simulink model "trimming"  (R2020a)
settings: Solver=VariableStepAuto  StartTime=0.0  StopTime=10.0  RelTol=1e-3
values from neighbouring files (symbols this model uses):
  g = 32.17    [PreLoadFcn.m]
  state0 = [IC.npos IC.epos IC.alt IC.q0 IC.q1 IC.q2 IC.q3  IC.p IC.q IC.r IC.alpha IC.beta IC.mu IC.Vt IC.chi IC.gamma]    [PreLoadFcn.m]
undefined symbols (not defined in the file or in its folder): Aactuator, ac, AeroCoeff, ft, kg, m, Newton, Raphson, s, slug
libraries: aerolibconvert2 x9, simulink x2
(part 1 of 2)
settings Model: Creator=User  LastModifiedBy=user

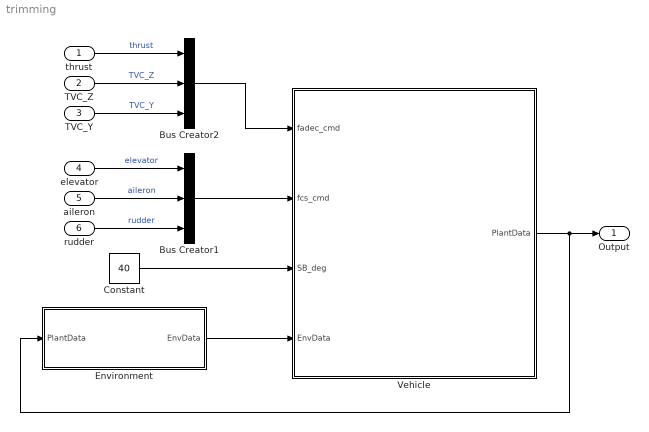
== system trimming ==
  thrust : Inport
  TVC_Z : Inport  Port=2
  TVC_Y : Inport  Port=3
  elevator : Inport  Port=4
  aileron : Inport  Port=5
  rudder : Inport  Port=6
  Bus Creator1 : BusCreator  Inputs=3
  Bus Creator2 : BusCreator  Inputs=3
  Constant : Constant  Value=40
  Environment : Subsystem
      mask Display:
      | image('aeroenvironment.bmp','center')
      | port_label('input',1,'PlantData')
      | port_label('output',1,'EnvData')
  Vehicle : Subsystem
  Output : Outport
  wires:
  Environment/1(EnvData) -> Vehicle/4(EnvData)
  Constant/1 -> Vehicle/3(" SB_deg")
  Vehicle/1(PlantData) -> Environment/1(PlantData), Output/1
  Bus Creator2/1 -> Vehicle/1(fadec_cmd)
  TVC_Y/1 -> Bus Creator2/3  "TVC_Y"
  TVC_Z/1 -> Bus Creator2/2  "TVC_Z"
  thrust/1 -> Bus Creator2/1  "thrust"
  elevator/1 -> Bus Creator1/1  "elevator"
  rudder/1 -> Bus Creator1/3  "rudder"
  aileron/1 -> Bus Creator1/2  "aileron"
  Bus Creator1/1 -> Vehicle/2(fcs_cmd)

== system trimming/Environment ==
  PlantData : Inport
  "ISP " : Subsystem
  end5 : Terminator
  end8 : Terminator
  end9 : Terminator
  gravity (ft/s^2) : Constant  Value=g
  Out Bus Element : Outport  PortName=EnvData  Element=P
  Out Bus Element1 : Outport  PortName=EnvData  Element=AirDensity
  Out Bus Element2 : Outport  PortName=EnvData  Element=qbar
  Out Bus Element3 : Outport  PortName=EnvData  Element=Mach
  Out Bus Element4 : Outport  PortName=EnvData  Element=g
  wires:
  "ISP "/7(mu) -> end9/1
  "ISP "/5(T(K)) -> end5/1
  "ISP "/6(g (m/s^2)) -> end8/1
  PlantData/1 -> "ISP "/1(PlantData)
  "ISP "/1(P(HPa)) -> Out Bus Element/1
  "ISP "/2(rho(kg/m^3)) -> Out Bus Element1/1
  "ISP "/3(qbar (lbf/ft^2)) -> Out Bus Element2/1
  "ISP "/4("Mach ") -> Out Bus Element3/1
  gravity (ft/s^2)/1 -> Out Bus Element4/1  "g"

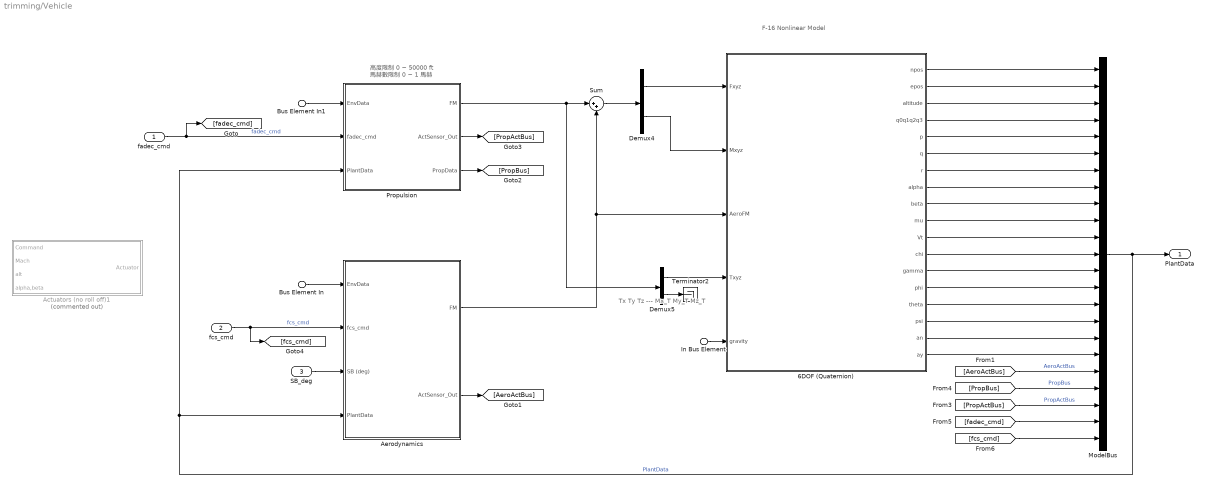
== system trimming/Vehicle ==
  note: F-16 Nonlinear Model
  note: Tx
      | Ty
      | Tz
      | ---
      | Mx_T
      | My_T
      | Mz_T
  note: 高度限制 0 ~ 50000 ft
      | 馬赫數限制 0 ~ 1 馬赫
  fadec_cmd : Inport
  fcs_cmd : Inport  Port=2
  " SB_deg" : Inport  Port=3
  Bus Element In : Inport  Port=4  PortName=EnvData
  Bus Element In1 : Inport  Port=4  PortName=EnvData
  In Bus Element : Inport  Port=4  PortName=EnvData  Element=g
  6DOF (Quaternion) : Subsystem
  Actuators (no roll off)1 : Subsystem  Commented=on
  Aerodynamics : Subsystem
  Demux4 : Demux  Outputs=[3, 3]
  Demux5 : Demux  Outputs=[3, 3]
  ModelBus : BusCreator  Inputs=23
  Propulsion : Subsystem
  Sum : Sum  Inputs=|++
  Terminator2 : Terminator
  PlantData : Outport
  wires:
  6DOF (Quaternion)/4(q0q1q2q3) -> ModelBus/4
  6DOF (Quaternion)/11(Vt) -> ModelBus/11
  6DOF (Quaternion)/3(altitude) -> ModelBus/3
  ModelBus/1 -> Aerodynamics/4(PlantData), Propulsion/3(PlantData), PlantData/1  "PlantData"
  6DOF (Quaternion)/1(npos) -> ModelBus/1
  6DOF (Quaternion)/2(epos) -> ModelBus/2
  " SB_deg"/1 -> Aerodynamics/3(" SB (deg)")
  Aerodynamics/1(FM) -> Sum/2, 6DOF (Quaternion)/3(AeroFM)
  Aerodynamics/2(ActSensor_Out) -> [AeroActBus]
  Propulsion/1(FM) -> Demux5/1, Sum/1
  fcs_cmd/1 -> [fcs_cmd], Aerodynamics/2(fcs_cmd)  "fcs_cmd"
  fadec_cmd/1 -> Propulsion/2(fadec_cmd), [fadec_cmd]  "fadec_cmd"
  Propulsion/2(ActSensor_Out) -> [PropActBus]
  Propulsion/3(PropData) -> [PropBus]
  Sum/1 -> Demux4/1
  Demux4/2 -> 6DOF (Quaternion)/2(Mxyz)
  Demux4/1 -> 6DOF (Quaternion)/1(Fxyz)
  Demux5/1 -> 6DOF (Quaternion)/4(Txyz)
  Demux5/2 -> Terminator2/1
  In Bus Element/1 -> 6DOF (Quaternion)/5(gravity)
  6DOF (Quaternion)/17(an) -> ModelBus/17
  6DOF (Quaternion)/18(ay) -> ModelBus/18
  6DOF (Quaternion)/5(p) -> ModelBus/5
  6DOF (Quaternion)/6(q) -> ModelBus/6
  6DOF (Quaternion)/7(r) -> ModelBus/7
  6DOF (Quaternion)/8(alpha) -> ModelBus/8
  6DOF (Quaternion)/9(beta) -> ModelBus/9
  6DOF (Quaternion)/10(mu) -> ModelBus/10
  6DOF (Quaternion)/12(chi) -> ModelBus/12
  6DOF (Quaternion)/13(gamma) -> ModelBus/13
  6DOF (Quaternion)/14(phi) -> ModelBus/14
  6DOF (Quaternion)/15(theta) -> ModelBus/15
  6DOF (Quaternion)/16(psi) -> ModelBus/16
  Bus Element In/1 -> Aerodynamics/1(EnvData)
  Bus Element In1/1 -> Propulsion/1(EnvData)
  [PropActBus] -> ModelBus/21  "PropActBus"
  [AeroActBus] -> ModelBus/19  "AeroActBus"
  [PropBus] -> ModelBus/20  "PropBus"
  [fadec_cmd] -> ModelBus/22
  [fcs_cmd] -> ModelBus/23

== system trimming/Environment/ISP  ==
  note: 1 T
      | 2 a (Speed of sound)
      | 3 P
      | 4 rho
      | 5 g
      | 6 mu (Coefficient of viscosity)
  In Bus Element : Inport  PortName=PlantData  Element=Vt
  In Bus Element1 : Inport  PortName=PlantData  Element=altitude
  Demux : Demux  Outputs=[1,1,1,1,1,1]
      settings: DisplayOption=none
  Density Conversion : aerolibconvert2/Density Conversion  IU=kg/m^3  OU=slug/ft^3
      settings: SourceProductBaseCode=AE
  Divide1 : Product  Inputs=*/
  Length Conversion : aerolibconvert2/Length Conversion  IU=ft  OU=m
  MATLAB Function : MATLAB Function  TreatAsAtomicUnit=on
  Product : Product
  Square : Math  Operator=square  SignedPower=on  SaturateOnIntegerOverflow=on
  Velocity Conversion : aerolibconvert2/Velocity Conversion  IU=m/s  OU=ft/s
  r2d1 : Gain  Gain=0.5  SaturateOnIntegerOverflow=on  OutDataTypeStr=Inherit: Same as input  ParamDataTypeStr=Inherit: Same as input
  r2d2 : Gain  Gain=-1  SaturateOnIntegerOverflow=on  OutDataTypeStr=Inherit: Same as input  ParamDataTypeStr=Inherit: Same as input
  P(HPa) : Outport  VectorParamsAs1DForOutWhenUnconnected=off
  rho(kg/m^3) : Outport  Port=2  VectorParamsAs1DForOutWhenUnconnected=off
  qbar (lbf/ft^2) : Outport  Port=3  VectorParamsAs1DForOutWhenUnconnected=off
  "Mach " : Outport  Port=4  VectorParamsAs1DForOutWhenUnconnected=off
  T(K) : Outport  Port=5  VectorParamsAs1DForOutWhenUnconnected=off
  g (m/s^2) : Outport  Port=6  VectorParamsAs1DForOutWhenUnconnected=off
  mu : Outport  Port=7  VectorParamsAs1DForOutWhenUnconnected=off
  wires:
  MATLAB Function/1(ISP_output) -> Demux/1
  Length Conversion/1 -> MATLAB Function/1(h)
  Velocity Conversion/1 -> Divide1/2
  Density Conversion/1 -> Product/2  "rho(slugs/ft^3)"
  Demux/4 -> Density Conversion/1, rho(kg/m^3)/1  "rho(kg/m^3)"
  Demux/2 -> Velocity Conversion/1  "a(m/s)"
  Demux/1 -> T(K)/1  "T(K)"
  Divide1/1 -> "Mach "/1
  Demux/5 -> g (m/s^2)/1  "g (m/s^2)"
  Demux/6 -> mu/1  "mu"
  Product/1 -> r2d1/1
  Square/1 -> Product/1
  In Bus Element/1 -> Divide1/1, Square/1  "Vt (ft/s)"
  Demux/3 -> P(HPa)/1  "P(Pa)"
  r2d2/1 -> Length Conversion/1  "H(ft)"
  r2d1/1 -> qbar (lbf/ft^2)/1  "qbar (lbf/ft^2)"
  In Bus Element1/1 -> r2d2/1

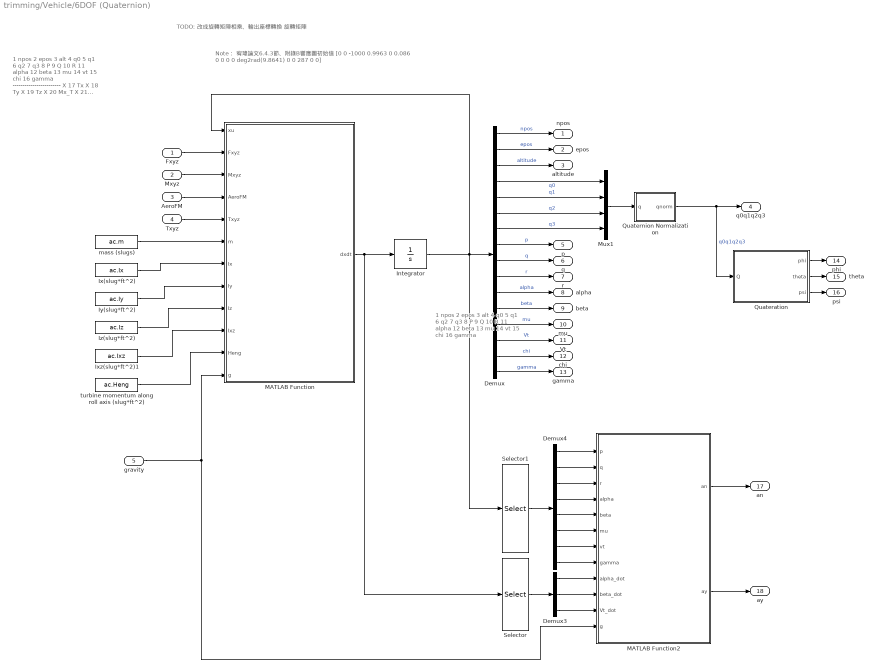
== system trimming/Vehicle/6DOF (Quaternion) ==
  note: TODO: 改成旋轉矩陣相乘、輸出座標轉換 旋轉矩陣
  note: 1 npos
      | 2 epos
      | 3 alt
      | 4 q0
      | 5 q1
      | 6 q2
      | 7 q3
      | 8 P
      | 9 Q
      | 10 R
      | 11 alpha
      | 12 beta
      | 13 mu
      | 14 vt
      | 15 chi
      | 16 gamma
      | ------------------------
      | X 17 Tx
      | X 18 Ty
      | X 19 Tz
      | X 20 Mx_T
      | X 21 My_T
      | X 22 Mz_T
      | X 23 T
      | --------------------
      | X 24 ele
      | X 25 ail
      | X 26 rud
      | -------------------
      | X 27 delta_z
      | X 28 delta_y
      | -----------------
      | X 29 qbar
      | -----------------
      | X 30 CXT
      | X 31 CYT
      | X 32 CZT
      | X 33 CLT
      | X 34 CMT
      | X 35 CNT
      | -----------------
      | X 36 lef
  note: 1 npos
      | 2 epos
      | 3 alt
      | 4 q0
      | 5 q1
      | 6 q2
      | 7 q3
      | 8 P
      | 9 Q
      | 10 R
      | 11 alpha
      | 12 beta
      | 13 mu
      | 14 vt
      | 15 chi
      | 16 gamma
  note: Note：
      |
      | 宥瑋論文6.4.3節、附錄B響應圖初始值
      | [0 0 -1000 0.9963 0 0.086 0  0 0 0 deg2rad(9.8641) 0 0 287 0 0]
  Fxyz : Inport
  Mxyz : Inport  Port=2
  AeroFM : Inport  Port=3
  Txyz : Inport  Port=4
  gravity : Inport  Port=5
  Demux : Demux  Outputs=16
      settings: DisplayOption=none
  Demux3 : Demux  Outputs=3
  Demux4 : Demux  Outputs=8
  Integrator : Integrator  InitialCondition=state0
  Ix(slug*ft^2) : Constant  Value=ac.Ix
  Ixz(slug*ft^2)1 : Constant  Value=ac.Ixz
  Iy(slug*ft^2) : Constant  Value=ac.Iy
  Iz(slug*ft^2) : Constant  Value=ac.Iz
  MATLAB Function : MATLAB Function  TreatAsAtomicUnit=on
  MATLAB Function2 : MATLAB Function  TreatAsAtomicUnit=on
  Mux1 : Mux  Inputs=[1,1,1,1]
  Quateration : MATLAB Function  TreatAsAtomicUnit=on
  Quaternion Normalization : Subsystem
  Selector : Selector  InputPortWidth=16  IndexOptions=Index vector (dialog)  Indices=[11 12 14]  OutputSizes=3
  Selector1 : Selector  InputPortWidth=16  IndexOptions=Index vector (dialog)  Indices=[8:14 16]  OutputSizes=3
  mass (slugs) : Constant  Value=ac.m
  turbine momentum along roll axis (slug*ft^2) : Constant  Value=ac.Heng
  npos : Outport  VectorParamsAs1DForOutWhenUnconnected=off
  epos : Outport  Port=2  VectorParamsAs1DForOutWhenUnconnected=off
  altitude : Outport  Port=3  VectorParamsAs1DForOutWhenUnconnected=off
  q0q1q2q3 : Outport  Port=4
  p : Outport  Port=5  VectorParamsAs1DForOutWhenUnconnected=off
  q : Outport  Port=6  VectorParamsAs1DForOutWhenUnconnected=off
  r : Outport  Port=7  VectorParamsAs1DForOutWhenUnconnected=off
  alpha : Outport  Port=8  VectorParamsAs1DForOutWhenUnconnected=off
  beta : Outport  Port=9  VectorParamsAs1DForOutWhenUnconnected=off
  mu : Outport  Port=10  VectorParamsAs1DForOutWhenUnconnected=off
  Vt : Outport  Port=11  VectorParamsAs1DForOutWhenUnconnected=off
  chi : Outport  Port=12  VectorParamsAs1DForOutWhenUnconnected=off
  gamma : Outport  Port=13  VectorParamsAs1DForOutWhenUnconnected=off
  phi : Outport  Port=14  VectorParamsAs1DForOutWhenUnconnected=off
  theta : Outport  Port=15  VectorParamsAs1DForOutWhenUnconnected=off
  psi : Outport  Port=16  VectorParamsAs1DForOutWhenUnconnected=off
  an : Outport  Port=17
  ay : Outport  Port=18
  wires:
  Demux/2 -> epos/1  "epos"
  Demux/3 -> altitude/1  "altitude"
  Integrator/1 -> MATLAB Function/1(xu), Selector1/1, Demux/1
  MATLAB Function/1(dxdt) -> Integrator/1, Selector/1
  Demux/1 -> npos/1  "npos"
  Demux/5 -> Mux1/2  "q1"
  Demux/4 -> Mux1/1  "q0"
  Demux/7 -> Mux1/4  "q3"
  Demux/6 -> Mux1/3  "q2"
  Demux/8 -> p/1  "p"
  Demux/9 -> q/1  "q"
  Demux/10 -> r/1  "r"
  Demux/11 -> alpha/1  "alpha"
  Demux/12 -> beta/1  "beta"
  Demux/13 -> mu/1  "mu"
  Demux/14 -> Vt/1  "Vt"
  Demux/15 -> chi/1  "chi"
  Demux/16 -> gamma/1  "gamma"
  Mux1/1 -> Quaternion Normalization/1(q)
  Quaternion Normalization/1(qnorm) -> q0q1q2q3/1, Quateration/1(Q)  "q0q1q2q3"
  AeroFM/1 -> MATLAB Function/4(AeroFM)
  Mxyz/1 -> MATLAB Function/3(Mxyz)
  Fxyz/1 -> MATLAB Function/2(Fxyz)
  Txyz/1 -> MATLAB Function/5(Txyz)
  gravity/1 -> MATLAB Function2/12(g), MATLAB Function/12(g)
  Ix(slug*ft^2)/1 -> MATLAB Function/7(Ix)
  Iy(slug*ft^2)/1 -> MATLAB Function/8(Iy)
  Iz(slug*ft^2)/1 -> MATLAB Function/9(Iz)
  Ixz(slug*ft^2)1/1 -> MATLAB Function/10(Ixz)
  turbine momentum along roll axis (slug*ft^2)/1 -> MATLAB Function/11(Heng)
  mass (slugs)/1 -> MATLAB Function/6(m)
  Quateration/1(phi) -> phi/1
  Quateration/2(theta) -> theta/1
  Quateration/3(psi) -> psi/1
  Selector/1 -> Demux3/1
  Demux3/1 -> MATLAB Function2/9(alpha_dot)
  Demux3/2 -> MATLAB Function2/10(beta_dot)
  Demux3/3 -> MATLAB Function2/11(Vt_dot)
  Selector1/1 -> Demux4/1
  Demux4/1 -> MATLAB Function2/1(p)
  Demux4/2 -> MATLAB Function2/2(q)
  Demux4/3 -> MATLAB Function2/3(r)
  Demux4/4 -> MATLAB Function2/4(alpha)
  Demux4/5 -> MATLAB Function2/5(beta)
  Demux4/6 -> MATLAB Function2/6(mu)
  Demux4/7 -> MATLAB Function2/7(vt)
  Demux4/8 -> MATLAB Function2/8(gamma)
  MATLAB Function2/1(an) -> an/1
  MATLAB Function2/2(ay) -> ay/1

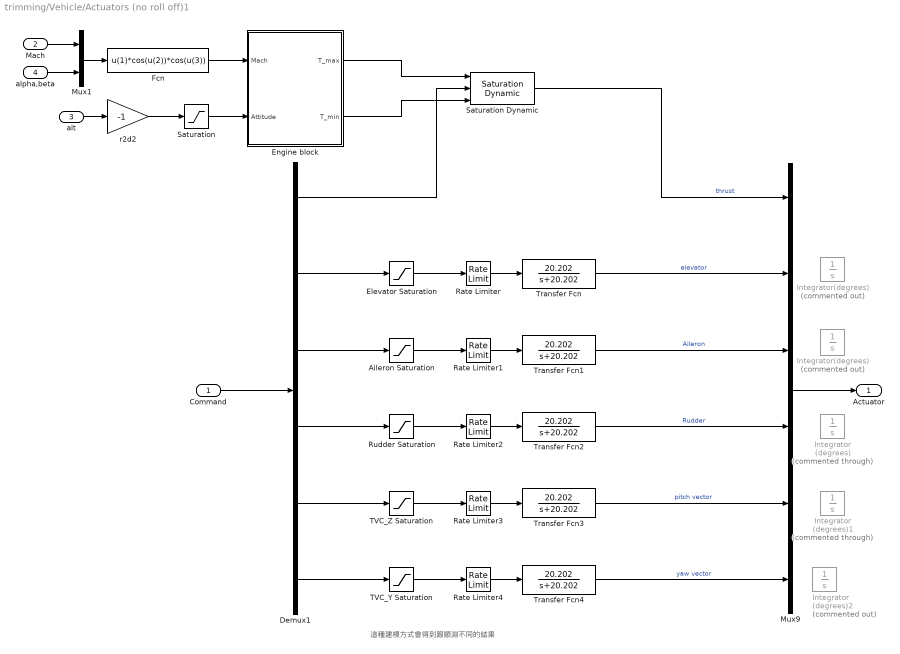
== system trimming/Vehicle/Actuators (no roll off)1 ==
  note: 這種建模方式會得到跟順淵不同的結果
  Command : Inport
  "Mach " : Inport  Port=2
  alt : Inport  Port=3
  alpha,beta : Inport  Port=4
  Aileron Saturation : Saturate  UpperLimit=21.5  LowerLimit=-21.5
  Demux1 : Demux  Outputs=6
  Elevator Saturation : Saturate  UpperLimit=25  LowerLimit=-25
  Engine block : Subsystem
  Fcn : Fcn  Expr=u(1)*cos(u(2))*cos(u(3))
  Integrator (degrees) : Integrator  Commented=through  InitialCondition=0.015206  UpperSaturationLimit=30  LowerSaturationLimit=-30
  Integrator (degrees)1 : Integrator  Commented=through  UpperSaturationLimit=30  LowerSaturationLimit=-30
  Integrator (degrees)2 : Integrator  Commented=on  UpperSaturationLimit=30  LowerSaturationLimit=-30
  Integrator(degrees) : Integrator  Commented=on  InitialCondition=-0.051516  UpperSaturationLimit=21.5  LowerSaturationLimit=-21.5
  "Integrator(degrees) " : Integrator  Commented=on  InitialCondition=-4.2454  UpperSaturationLimit=25  LowerSaturationLimit=-25
  Mux1 : Mux  Inputs=2
  Mux9 : Mux  Inputs=6
  Rate Limiter : RateLimiter  RisingSlewLimit=+60  FallingSlewLimit=-60  SampleTimeMode=inherited
  Rate Limiter1 : RateLimiter  RisingSlewLimit=+80  FallingSlewLimit=-80  SampleTimeMode=inherited
  Rate Limiter2 : RateLimiter  RisingSlewLimit=+120  FallingSlewLimit=-120  SampleTimeMode=inherited
  Rate Limiter3 : RateLimiter  RisingSlewLimit=+60  FallingSlewLimit=-60  SampleTimeMode=inherited
  Rate Limiter4 : RateLimiter  RisingSlewLimit=+60  FallingSlewLimit=-60  SampleTimeMode=inherited
  Rudder Saturation : Saturate  UpperLimit=30  LowerLimit=-30
  Saturation : Saturate  UpperLimit=50000  LowerLimit=0
  Saturation Dynamic : simulink/Discontinuities/Saturation Dynamic  OutMin=[]  OutMax=[]  OutDataTypeStr=Inherit: Same as second input  OutDataType=fixdt(1, 16)  OutScaling=2^-10  DoSatur=off
  TVC_Y Saturation : Saturate  UpperLimit=15  LowerLimit=-15
  TVC_Z Saturation : Saturate  UpperLimit=15  LowerLimit=-15
  Transfer Fcn{,1..4} (5 alike) : TransferFcn  Numerator=[20.202]  Denominator=[1 20.202]
  r2d2 : Gain  Gain=-1  SaturateOnIntegerOverflow=on  OutDataTypeStr=Inherit: Same as input  ParamDataTypeStr=Inherit: Same as input
  Actuator : Outport  VectorParamsAs1DForOutWhenUnconnected=off
  wires:
  Mux9/1 -> Actuator/1
  Command/1 -> Demux1/1
  Transfer Fcn/1 -> Mux9/2  "elevator"
  Transfer Fcn1/1 -> Mux9/3  "Aileron"
  Transfer Fcn2/1 -> Mux9/4  "Rudder"
  Saturation Dynamic/1 -> Mux9/1  "thrust"
  Transfer Fcn4/1 -> Mux9/6  "yaw vector"
  Transfer Fcn3/1 -> Mux9/5  "pitch vector"
  r2d2/1 -> Saturation/1
  alt/1 -> r2d2/1
  Demux1/1 -> Saturation Dynamic/2
  "Mach "/1 -> Mux1/1
  alpha,beta/1 -> Mux1/2
  Mux1/1 -> Fcn/1
  Fcn/1 -> Engine block/1(Mach)
  Saturation/1 -> Engine block/2(Attitude)
  Engine block/2(T_min) -> Saturation Dynamic/3
  Engine block/1(T_max) -> Saturation Dynamic/1
  Demux1/2 -> Elevator Saturation/1
  Elevator Saturation/1 -> Rate Limiter/1
  Demux1/3 -> Aileron Saturation/1
  Aileron Saturation/1 -> Rate Limiter1/1
  Demux1/4 -> Rudder Saturation/1
  Rudder Saturation/1 -> Rate Limiter2/1
  Demux1/5 -> TVC_Z Saturation/1
  TVC_Z Saturation/1 -> Rate Limiter3/1
  Demux1/6 -> TVC_Y Saturation/1
  TVC_Y Saturation/1 -> Rate Limiter4/1
  Rate Limiter/1 -> Transfer Fcn/1
  Rate Limiter1/1 -> Transfer Fcn1/1
  Rate Limiter2/1 -> Transfer Fcn2/1
  Rate Limiter3/1 -> Transfer Fcn3/1
  Rate Limiter4/1 -> Transfer Fcn4/1

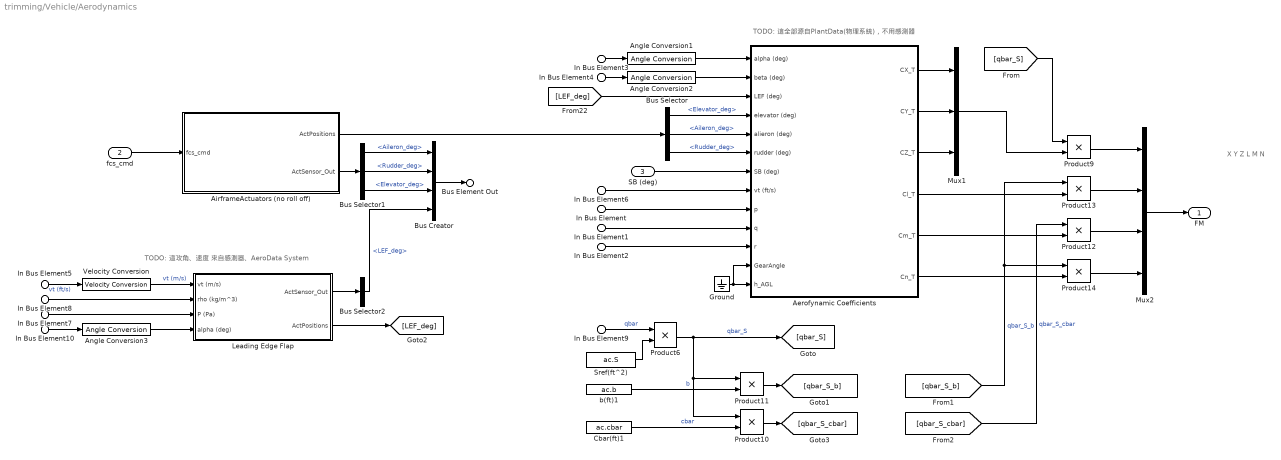
== system trimming/Vehicle/Aerodynamics ==
  note: TODO: 這全部源自PlantData(物理系統)，不用感測器
  note: TODO: 這攻角、速度 來自感測器、AeroData System
  note: X
      | Y
      | Z
      | L
      | M
      | N
  In Bus Element7 : Inport  PortName=EnvData  Element=P
  In Bus Element8 : Inport  PortName=EnvData  Element=AirDensity
  In Bus Element9 : Inport  PortName=EnvData  Element=qbar
  fcs_cmd : Inport  Port=2
  " SB (deg)" : Inport  Port=3
  In Bus Element : Inport  Port=4  PortName=PlantData  Element=p
  In Bus Element1 : Inport  Port=4  PortName=PlantData  Element=q
  In Bus Element2 : Inport  Port=4  PortName=PlantData  Element=r
  In Bus Element3 : Inport  Port=4  PortName=PlantData  Element=alpha
  In Bus Element10 : Inport  Port=4  PortName=PlantData  Element=alpha
  In Bus Element4 : Inport  Port=4  PortName=PlantData  Element=beta
  In Bus Element6 : Inport  Port=4  PortName=PlantData  Element=Vt
  In Bus Element5 : Inport  Port=4  PortName=PlantData  Element=Vt
  Aerofynamic Coefficients : Subsystem
  AirframeActuators (no roll off) : Subsystem
  Angle Conversion1 : aerolibconvert2/Angle Conversion  IU=rad  OU=deg
  Angle Conversion2 : aerolibconvert2/Angle Conversion  IU=rad  OU=deg
  Angle Conversion3 : aerolibconvert2/Angle Conversion  IU=rad  OU=deg
  Bus Creator : BusCreator  Inputs=4
  Bus Selector : BusSelector  OutputSignals=Elevator_deg,Aileron_deg,Rudder_deg
  Bus Selector1 : BusSelector  OutputSignals=Aileron_deg,Rudder_deg,Elevator_deg
  Bus Selector2 : BusSelector  OutputSignals=LEF_deg
  Cbar(ft)1 : Constant  Value=ac.cbar
  Ground : Ground
  Leading Edge Flap : Subsystem
  Mux1 : Mux  Inputs=3
  Mux2 : Mux
  Product{6,9..14} (7 alike) : Product
  Sref(ft^2) : Constant  Value=ac.S
  Velocity Conversion : aerolibconvert2/Velocity Conversion  IU=ft/s  OU=m/s
  b(ft)1 : Constant  Value=ac.b
  FM : Outport
  Bus Element Out : Outport  Port=2  PortName=ActSensor_Out
  wires:
  Bus Selector/2 -> Aerofynamic Coefficients/5(alieron (deg))  "<Aileron_deg>"
  " SB (deg)"/1 -> Aerofynamic Coefficients/7(SB (deg))
  In Bus Element1/1 -> Aerofynamic Coefficients/10(q)
  In Bus Element/1 -> Aerofynamic Coefficients/9(p)
  Bus Selector/3 -> Aerofynamic Coefficients/6(rudder (deg))  "<Rudder_deg>"
  Angle Conversion2/1 -> Aerofynamic Coefficients/2(beta (deg))
  Angle Conversion1/1 -> Aerofynamic Coefficients/1(alpha (deg))
  In Bus Element2/1 -> Aerofynamic Coefficients/11(r)
  [LEF_deg] -> Aerofynamic Coefficients/3(LEF (deg))
  Bus Selector/1 -> Aerofynamic Coefficients/4(elevator (deg))  "<Elevator_deg>"
  Ground/1 -> Aerofynamic Coefficients/13(h_AGL), Aerofynamic Coefficients/12(GearAngle)
  Mux1/1 -> Product9/2
  [qbar_S] -> Product9/1
  Aerofynamic Coefficients/6(Cn_T) -> Product14/2
  Aerofynamic Coefficients/5(Cm_T) -> Product12/2
  [qbar_S_cbar] -> Product12/1  "qbar_S_cbar"
  Aerofynamic Coefficients/4(Cl_T) -> Product13/2
  [qbar_S_b] -> Product13/1, Product14/1  "qbar_S_b"
  Aerofynamic Coefficients/1(CX_T) -> Mux1/1
  Aerofynamic Coefficients/2(CY_T) -> Mux1/2
  Aerofynamic Coefficients/3(CZ_T) -> Mux1/3
  Product13/1 -> Mux2/2
  Product12/1 -> Mux2/3
  Product14/1 -> Mux2/4
  Product9/1 -> Mux2/1
  Mux2/1 -> FM/1
  Sref(ft^2)/1 -> Product6/2
  b(ft)1/1 -> Product11/2  "b"
  Product11/1 -> [qbar_S_b]
  Product10/1 -> [qbar_S_cbar]
  Cbar(ft)1/1 -> Product10/2  "cbar"
  In Bus Element9/1 -> Product6/1  "qbar"
  Product6/1 -> Product11/1, Product10/1, [qbar_S]  "qbar_S"
  Leading Edge Flap/2(ActPositions) -> [LEF_deg]
  Velocity Conversion/1 -> Leading Edge Flap/1(vt (m/s))  "vt (m/s)"
  In Bus Element6/1 -> Aerofynamic Coefficients/8(vt (ft/s))
  In Bus Element8/1 -> Leading Edge Flap/2(rho (kg/m^3))
  In Bus Element7/1 -> Leading Edge Flap/3(P (Pa))
  AirframeActuators (no roll off)/1(ActPositions) -> Bus Selector/1
  fcs_cmd/1 -> AirframeActuators (no roll off)/1(fcs_cmd)
  In Bus Element3/1 -> Angle Conversion1/1
  In Bus Element4/1 -> Angle Conversion2/1
  In Bus Element5/1 -> Velocity Conversion/1  "vt (ft/s)"
  AirframeActuators (no roll off)/2(ActSensor_Out) -> Bus Selector1/1
  Bus Selector1/1 -> Bus Creator/1  "<Aileron_deg>"
  Bus Selector1/2 -> Bus Creator/2  "<Rudder_deg>"
  Bus Selector1/3 -> Bus Creator/3  "<Elevator_deg>"
  Bus Creator/1 -> Bus Element Out/1
  In Bus Element10/1 -> Angle Conversion3/1
  Angle Conversion3/1 -> Leading Edge Flap/4(alpha (deg))
  Leading Edge Flap/1(ActSensor_Out) -> Bus Selector2/1
  Bus Selector2/1 -> Bus Creator/4  "<LEF_deg>"

== system trimming/Vehicle/Propulsion ==
  note: 高度限制 0 ~ 50000 ft
      | 馬赫數限制 0 ~ 1 馬赫
  note: Thrust Vector Nozzle Module 向量噴嘴模組
  note: Commands_TVC_Z_pitch
      | Commands_TVC_Y_yaw
  note: Inlet 進氣道
  In Bus Element1 : Inport  PortName=EnvData  Element=Mach
  Bus Element In2 : Inport  Port=2  PortName=fadec_cmd
  In Bus Element2 : Inport  Port=2  PortName=fadec_cmd  Element=thrust
  Bus Element In1 : Inport  Port=3  PortName=PlantData  Element=beta
  Bus Element In : Inport  Port=3  PortName=PlantData  Element=alpha
  In Bus Element : Inport  Port=3  PortName=PlantData  Element=altitude
  Actuators : Subsystem
  Afterburning Turbofan Jet Engine : Subsystem
  Cos : Trigonometry  Operator=cos
  Cos1 : Trigonometry  Operator=cos
  Product : Product  Inputs=3
  Saturation Dynamic : simulink/Discontinuities/Saturation Dynamic  OutMin=[]  OutMax=[]  OutDataTypeStr=Inherit: Same as second input  OutDataType=fixdt(1, 16)  OutScaling=2^-10  DoSatur=off
  Thrust Vector Nozzle ZY : Subsystem
  nozzle position : Constant  Value=ac.lt
  r2d1 : Gain  Gain=-1  SaturateOnIntegerOverflow=on  OutDataTypeStr=Inherit: Same as input  ParamDataTypeStr=Inherit: Same as input
  FM : Outport
  Bus Element Out : Outport  Port=2  PortName=ActSensor_Out
  Bus Element Out1 : Outport  Port=3  PortName=PropData  Element=Tx
  Bus Element Out2 : Outport  Port=3  PortName=PropData  Element=Ty
  Bus Element Out3 : Outport  Port=3  PortName=PropData  Element=Tz
  Bus Element Out4 : Outport  Port=3  PortName=PropData  Element=T
  wires:
  Actuators/2(ActSensor_Out) -> Bus Element Out/1
  nozzle position/1 -> Thrust Vector Nozzle ZY/3(" lt")
  Actuators/1(ActPositions) -> Thrust Vector Nozzle ZY/2(Actuator (deg))
  Thrust Vector Nozzle ZY/1(FM) -> FM/1
  Product/1 -> Afterburning Turbofan Jet Engine/1(Mach)
  r2d1/1 -> Afterburning Turbofan Jet Engine/2(H (ft))
  Cos/1 -> Product/2
  Saturation Dynamic/1 -> Bus Element Out4/1, Thrust Vector Nozzle ZY/1(T)  "Thrust (lbf)"
  Bus Element In1/1 -> Cos1/1  "beta (rad)"
  Afterburning Turbofan Jet Engine/2(T_min) -> Saturation Dynamic/3
  In Bus Element1/1 -> Product/1
  Cos1/1 -> Product/3
  Bus Element In/1 -> Cos/1  "alpha (rad)"
  Afterburning Turbofan Jet Engine/1(T_max) -> Saturation Dynamic/1
  In Bus Element/1 -> r2d1/1
  In Bus Element2/1 -> Saturation Dynamic/2  "Commands_Tc"
  Bus Element In2/1 -> Actuators/1(Commands)
  Thrust Vector Nozzle ZY/2(Tx) -> Bus Element Out1/1
  Thrust Vector Nozzle ZY/3(Ty) -> Bus Element Out2/1
  Thrust Vector Nozzle ZY/4(Tz) -> Bus Element Out3/1

== system trimming/Vehicle/6DOF (Quaternion)/Quaternion Normalization ==
  q : Inport  PortDimensions=4
  Product : Product  Inputs=*/  InputSameDT=on  RndMeth=Zero  SaturateOnIntegerOverflow=on  OutDataTypeStr=Inherit: Same as first input
  Square : Math  Operator=square  SignedPower=on  SaturateOnIntegerOverflow=on
  Square Root : Sqrt  Operator=signedSqrt  AlgorithmType=Newton-Raphson  SaturateOnIntegerOverflow=on
  Sum : Sum  Inputs=1  InputSameDT=on  SaturateOnIntegerOverflow=on  OutDataTypeStr=Inherit: Same as first input
  qnorm : Outport  VectorParamsAs1DForOutWhenUnconnected=off
  wires:
  Product/1 -> qnorm/1
  Square Root/1 -> Product/2
  Square/1 -> Sum/1
  Sum/1 -> Square Root/1
  q/1 -> Product/1, Square/1

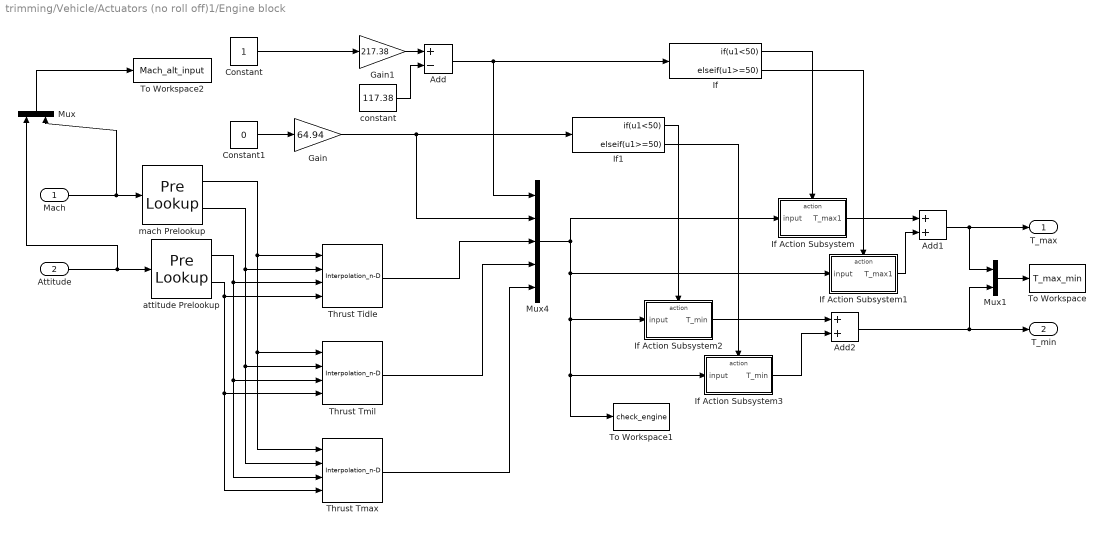
== system trimming/Vehicle/Actuators (no roll off)1/Engine block ==
  Mach : Inport
  Attitude : Inport  Port=2
  Add : Sum  Inputs=+-
  Add1 : Sum
  Add2 : Sum
  Constant : Constant
  Constant1 : Constant  Value=0
  Gain : Gain  Gain=64.94
  Gain1 : Gain  Gain=217.38
  If : If  IfExpression=u1<50  ElseIfExpressions=u1>=50  ShowElse=off
  If Action Subsystem : Subsystem  TreatAsAtomicUnit=on
  If Action Subsystem1 : Subsystem  TreatAsAtomicUnit=on
  If Action Subsystem2 : Subsystem  TreatAsAtomicUnit=on
  If Action Subsystem3 : Subsystem  TreatAsAtomicUnit=on
  If1 : If  IfExpression=u1<50  ElseIfExpressions=u1>=50  ShowElse=off
  Mux : Mux  Inputs=2
  Mux1 : Mux  Inputs=2
  Mux4 : Mux  Inputs=5
  Thrust Tidle : Interpolation_n-D  Table=|  InternalRulePriority=Speed
      | [1060	670	880	1140	1500	1860
      | 635	425	690	1010	1330	1700
      | 60	25	345	755	1130	1525
      | -1020	-710	-300	350	910	1360
      | -2700	-1900	-1300	-247	600	1100
      | -3600	-1400	-595	-342	-200	700]
  Thrust Tmax : Interpolation_n-D  Table=reshape([20000,21420,22700,24240,26070,28886,15000,15700,16860,18910,21075,23319,10800,11225,12250,13760,15975,18300,7000,7323,8154,9285,11115,13484,4000,4435,5000,5700,6860,8642,2500,2600,2835,3215,3950,5057],6,6)  InternalRulePriority=Speed
  Thrust Tmil : Interpolation_n-D  Table=|  InternalRulePriority=Speed
      | [12680	9150	6200	3950	2450	1400
      | 12680	9150	6313	4040	2470	1400
      | 12610	9312	6610	4290	2600	1560
      | 12640	9839	7090	4660	2840	1660
      | 12390	10176	7750	5320	3250	1930
      | 11680	9848	8050	6100	3800	2310]
  To Workspace : ToWorkspace  VariableName=T_max_min  SaveFormat=Timeseries  SampleTime=-1
  To Workspace1 : ToWorkspace  VariableName=check_engine  SaveFormat=Timeseries  SampleTime=-1
  To Workspace2 : ToWorkspace  VariableName=Mach_alt_input  SaveFormat=Timeseries  SampleTime=-1
  attitude Prelookup : PreLookup  BreakpointsData=[0,10000,20000,30000,40000,50000]  IndexSearchMethod=Linear search  BeginIndexSearchUsingPreviousIndexResult=on  DiagnosticForOutOfRangeInput=Warning
  constant : Constant  Value=117.38
  mach Prelookup : PreLookup  BreakpointsData=[0,0.2,0.4,0.6,0.8,1]  IndexSearchMethod=Linear search  BeginIndexSearchUsingPreviousIndexResult=on  DiagnosticForOutOfRangeInput=Warning
  T_max : Outport  VectorParamsAs1DForOutWhenUnconnected=off
  T_min : Outport  Port=2  VectorParamsAs1DForOutWhenUnconnected=off
  wires:
  Mach/1 -> Mux/2, mach Prelookup/1
  Attitude/1 -> attitude Prelookup/1, Mux/1
  Add2/1 -> T_min/1, Mux1/2
  Add1/1 -> T_max/1, Mux1/1
  attitude Prelookup/2 -> Thrust Tidle/4, Thrust Tmil/4, Thrust Tmax/4
  Mux1/1 -> To Workspace/1
  Thrust Tmil/1 -> Mux4/4
  Mux/1 -> To Workspace2/1
  Gain1/1 -> Add/1
  If Action Subsystem1/1(T_max1) -> Add1/2
  Constant/1 -> Gain1/1
  mach Prelookup/1 -> Thrust Tidle/1, Thrust Tmil/1, Thrust Tmax/1
  If/2 -> If Action Subsystem1/Action
  If1/2 -> If Action Subsystem3/Action
  If Action Subsystem3/1(T_min) -> Add2/2
  If Action Subsystem2/1(T_min) -> Add2/1
  If1/1 -> If Action Subsystem2/Action
  Gain/1 -> Mux4/2, If1/1
  If Action Subsystem/1(T_max1) -> Add1/1
  Thrust Tmax/1 -> Mux4/5
  mach Prelookup/2 -> Thrust Tidle/2, Thrust Tmil/2, Thrust Tmax/2
  Thrust Tidle/1 -> Mux4/3
  If/1 -> If Action Subsystem/Action
  Add/1 -> Mux4/1, If/1
  constant/1 -> Add/2
  Mux4/1 -> If Action Subsystem1/1("input "), If Action Subsystem2/1("input "), If Action Subsystem3/1("input "), To Workspace1/1, If Action Subsystem/1("input ")
  Constant1/1 -> Gain/1
  attitude Prelookup/1 -> Thrust Tidle/3, Thrust Tmil/3, Thrust Tmax/3

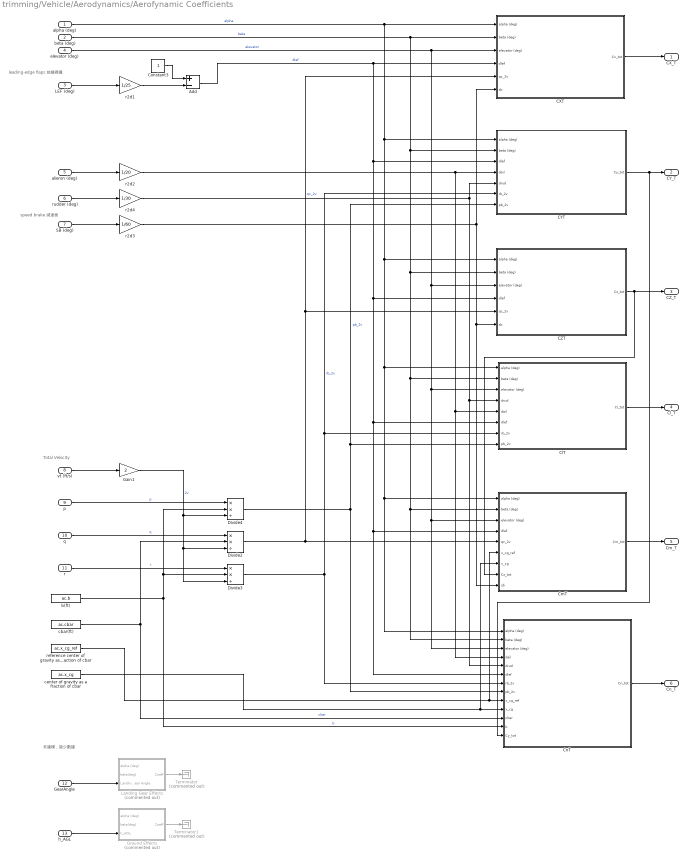
== system trimming/Vehicle/Aerodynamics/Aerofynamic Coefficients ==
  note: Total Velocity
  note: 未建模，缺少數據
  note: speed brake
      | 減速板
  note: leading-edge flaps
      | 前緣襟翼
  alpha (deg) : Inport
  beta (deg) : Inport  Port=2
  LEF (deg) : Inport  Port=3
  elevator (deg) : Inport  Port=4
  alieron (deg) : Inport  Port=5
  rudder (deg) : Inport  Port=6
  SB (deg) : Inport  Port=7
  vt (ft/s) : Inport  Port=8
  p : Inport  Port=9
  q : Inport  Port=10
  r : Inport  Port=11
  GearAngle : Inport  Port=12
  h_AGL : Inport  Port=13
  Add : Sum  Inputs=+-
  CXT : Subsystem
  CYT : Subsystem
  CZT : Subsystem
  ClT : Subsystem
  CmT : Subsystem
  CnT : Subsystem
  Constant3 : Constant
  Divide2 : Product  Inputs=**/
  Divide3 : Product  Inputs=**/
  Divide4 : Product  Inputs=**/
  Gain1 : Gain  Gain=2
  Ground Effects : Subsystem  Commented=on
  Landing Gear Effects : Subsystem  Commented=on
  Terminator : Terminator  Commented=on
  Terminator1 : Terminator  Commented=on
  b(ft) : Constant  Value=ac.b
  cbar(ft) : Constant  Value=ac.cbar
  center of gravity as a fraction of cbar : Constant  Value=ac.x_cg
  r2d1 : Gain  Gain=1/25  SaturateOnIntegerOverflow=on  OutDataTypeStr=Inherit: Same as input  ParamDataTypeStr=Inherit: Same as input
  r2d2 : Gain  Gain=1/20  SaturateOnIntegerOverflow=on  OutDataTypeStr=Inherit: Same as input  ParamDataTypeStr=Inherit: Same as input
  r2d3 : Gain  Gain=1/60  SaturateOnIntegerOverflow=on  OutDataTypeStr=Inherit: Same as input  ParamDataTypeStr=Inherit: Same as input
  r2d4 : Gain  Gain=1/30  SaturateOnIntegerOverflow=on  OutDataTypeStr=Inherit: Same as input  ParamDataTypeStr=Inherit: Same as input
  reference center of gravity as a fraction of cbar : Constant  Value=ac.x_cg_ref
  CX_T : Outport  VectorParamsAs1DForOutWhenUnconnected=off
  CY_T : Outport  Port=2  VectorParamsAs1DForOutWhenUnconnected=off
  CZ_T : Outport  Port=3  VectorParamsAs1DForOutWhenUnconnected=off
  Cl_T : Outport  Port=4  VectorParamsAs1DForOutWhenUnconnected=off
  Cm_T : Outport  Port=5  VectorParamsAs1DForOutWhenUnconnected=off
  Cn_T : Outport  Port=6  VectorParamsAs1DForOutWhenUnconnected=off
  wires:
  alpha (deg)/1 -> ClT/1(alpha (deg)), CnT/1(alpha (deg)), CmT/1(alpha (deg)), CZT/1(alpha (deg)), CYT/1(alpha (deg)), CXT/1(alpha (deg))  "alpha"
  beta (deg)/1 -> ClT/2(beta (deg)), CnT/2(beta (deg)), CmT/2(beta (deg)), CZT/2(beta (deg)), CYT/2(beta (deg)), CXT/2("beta (deg) ")  "beta"
  elevator (deg)/1 -> ClT/3(elevator (deg)), CnT/3(elevator (deg)), CmT/3(elevator (deg)), CZT/3(elevator (deg)), CXT/3(elevator (deg))  "elevator"
  vt (ft/s)/1 -> Gain1/1
  q/1 -> Divide2/1  "q"
  r/1 -> Divide3/1  "r"
  Divide2/1 -> CXT/5(qc_2v), CZT/5(qc_2v), CmT/5(qc_2v)  "qc_2v"
  Divide3/1 -> CYT/6(rb_2v), ClT/7(rb_2v), CnT/7(rb_2v)  "rb_2v"
  Divide4/1 -> CYT/7(pb_2v), ClT/8(pb_2v), CnT/8(pb_2v)  "pb_2v"
  b(ft)/1 -> CnT/12(b), Divide3/2, Divide4/2  "b"
  cbar(ft)/1 -> CnT/11(cbar), Divide2/2  "cbar"
  reference center of gravity as a fraction of cbar/1 -> CmT/6(x_cg_ref), CnT/9(x_cg_ref)
  center of gravity as a fraction of cbar/1 -> CmT/7(x_cg), CnT/10(x_cg)
  CZT/1(Cz_tot) -> CmT/8(Cz_tot), CZ_T/1
  CYT/1(Cy_tot) -> CnT/13(Cy_tot), CY_T/1
  CXT/1(Cx_tot) -> CX_T/1
  ClT/1(Cl_tot) -> Cl_T/1
  CmT/1(Cm_tot) -> Cm_T/1
  CnT/1(Cn_tot) -> Cn_T/1
  Add/1 -> CmT/4(dlef), CnT/6(dlef), ClT/6(dlef), CZT/4(dlef), CYT/3(dlef), CXT/4(dlef)  "dlef"
  alieron (deg)/1 -> r2d2/1
  rudder (deg)/1 -> r2d4/1
  SB (deg)/1 -> r2d3/1
  r2d1/1 -> Add/2
  Constant3/1 -> Add/1
  LEF (deg)/1 -> r2d1/1
  Gain1/1 -> Divide4/3, Divide3/3, Divide2/3  "2v"
  p/1 -> Divide4/1  "p"
  r2d3/1 -> CZT/6(sb), CmT/9(sb), CXT/6(sb)
  r2d2/1 -> CnT/4(dail), ClT/5(dail), CYT/4(dail)
  r2d4/1 -> CYT/5(drud), CnT/5(drud), ClT/4(drud)
  GearAngle/1 -> Landing Gear Effects/3(Landing Gear Angle)
  h_AGL/1 -> Ground Effects/3(h_AGL)
  Landing Gear Effects/1(Coeff) -> Terminator/1
  Ground Effects/1(Coeff) -> Terminator1/1

== system trimming/Vehicle/Aerodynamics/AirframeActuators (no roll off) ==
  note: 初始值全部等於0和非0
      | 會影響模擬結果
  In Bus Element : Inport  PortName=fcs_cmd  Element=elevator
  In Bus Element1 : Inport  PortName=fcs_cmd  Element=aileron
  In Bus Element2 : Inport  PortName=fcs_cmd  Element=rudder
  Aileron Saturation : Saturate  UpperLimit=Aactuator.aileron.AngleLimitUpper  LowerLimit=Aactuator.aileron.AngleLimitLower
  Elevator Saturation : Saturate  UpperLimit=Aactuator.elevator.AngleLimitUpper  LowerLimit=Aactuator.elevator.AngleLimitLower
  Gain : Gain  Gain=20.202  SaturateOnIntegerOverflow=on  OutDataTypeStr=Inherit: Same as input  ParamDataTypeStr=Inherit: Same as input
  Gain1 : Gain  Gain=20.202  SaturateOnIntegerOverflow=on  OutDataTypeStr=Inherit: Same as input  ParamDataTypeStr=Inherit: Same as input
  Gain2 : Gain  Gain=20.202  SaturateOnIntegerOverflow=on  OutDataTypeStr=Inherit: Same as input  ParamDataTypeStr=Inherit: Same as input
  Rate Saturation : Saturate  UpperLimit=Aactuator.elevator.RateLimitUpper  LowerLimit=Aactuator.elevator.RateLimitLower
  Rate Saturation1 : Saturate  UpperLimit=Aactuator.aileron.RateLimitUpper  LowerLimit=Aactuator.aileron.RateLimitLower
  Rate Saturation2 : Saturate  UpperLimit=Aactuator.rudder.RateLimitUpper  LowerLimit=Aactuator.rudder.RateLimitLower
  Rudder Saturation : Saturate  UpperLimit=Aactuator.rudder.AngleLimitUpper  LowerLimit=Aactuator.rudder.AngleLimitLower
  Sum : Sum  Inputs=|+-  InputSameDT=on  SaturateOnIntegerOverflow=on  OutDataTypeStr=Inherit: Same as first input
  Sum1 : Sum  Inputs=|+-  InputSameDT=on  SaturateOnIntegerOverflow=on  OutDataTypeStr=Inherit: Same as first input
  Sum2 : Sum  Inputs=|+-  InputSameDT=on  SaturateOnIntegerOverflow=on  OutDataTypeStr=Inherit: Same as first input
  aileron Integrator(degrees) : Integrator  InitialCondition=Aactuator.aileron.IntegratorInitial  UpperSaturationLimit=21.5  LowerSaturationLimit=-21.5
  "elevator Integrator(degrees) " : Integrator  InitialCondition=Aactuator.elevator.IntegratorInitial  UpperSaturationLimit=25  LowerSaturationLimit=-25
  rudder Integrator (degrees) : Integrator  InitialCondition=Aactuator.rudder.IntegratorInitial  UpperSaturationLimit=30  LowerSaturationLimit=-30
  Out Bus Element : Outport  PortName=ActPositions  Element=Aileron_deg
  Out Bus Element1 : Outport  PortName=ActPositions  Element=Rudder_deg
  Out Bus Element4 : Outport  PortName=ActPositions  Element=Elevator_deg
  Out Bus Element2 : Outport  Port=2  PortName=ActSensor_Out  Element=Aileron_deg
  Out Bus Element3 : Outport  Port=2  PortName=ActSensor_Out  Element=Rudder_deg
  Out Bus Element5 : Outport  Port=2  PortName=ActSensor_Out  Element=Elevator_deg
  wires:
  Gain/1 -> Rate Saturation/1
  Gain1/1 -> Rate Saturation1/1
  In Bus Element/1 -> Elevator Saturation/1  "cmd_elevator_deg"
  Rudder Saturation/1 -> Sum2/1
  Rate Saturation/1 -> "elevator Integrator(degrees) "/1
  aileron Integrator(degrees)/1 -> Out Bus Element2/1, Out Bus Element/1, Sum1/2  "Aileron_deg"
  Rate Saturation1/1 -> aileron Integrator(degrees)/1
  Gain2/1 -> Rate Saturation2/1
  Sum1/1 -> Gain1/1
  Elevator Saturation/1 -> Sum/1
  rudder Integrator (degrees)/1 -> Out Bus Element3/1, Out Bus Element1/1, Sum2/2  "Rudder_deg"
  Rate Saturation2/1 -> rudder Integrator (degrees)/1
  Aileron Saturation/1 -> Sum1/1
  Sum/1 -> Gain/1
  Sum2/1 -> Gain2/1
  "elevator Integrator(degrees) "/1 -> Sum/2, Out Bus Element5/1, Out Bus Element4/1  "Elevator_deg"
  In Bus Element1/1 -> Aileron Saturation/1  "cmd_aileron_deg"
  In Bus Element2/1 -> Rudder Saturation/1  "cmd_rudder_deg"

== system trimming/Vehicle/Aerodynamics/Leading Edge Flap ==
  note: $\delta_{LEF} =1.38\frac{2s+7.25}{s+7.25}\alpha -9.05\frac{\bar{q} }{p_s }+1.45$
      | $\alpha$ 的單位：deg
      | $\bar{q}$ 是動壓， $p_s$ 是靜壓，兩者單位要一致 (公制：1Pa = 1 $N/m^2$ = 1 $\mathrm{kg}/\left(m{\cdot s}^2 \right)$ ；英制：1psf = 1 $\mathrm{lbf}/{\mathrm{ft}}^2$ = 1 $\mathrm{slugs}/\left(\mathrm{ft}\cdot s^2 \right)$ )
  vt (m/s) : Inport
  rho (kg/m^3) : Inport  Port=2
  P (Pa) : Inport  Port=3
  alpha (deg) : Inport  Port=4
  Divide1 : Product  Inputs=*/
  Divide2 : Product  Inputs=**
  Gain2 : Gain  Gain=1.38  SaturateOnIntegerOverflow=on  OutDataTypeStr=Inherit: Same as input  ParamDataTypeStr=Inherit: Same as input
  LEF Rate Limiter : RateLimiter  RisingSlewLimit=Aactuator.LEF.RateLimitUpper  FallingSlewLimit=Aactuator.LEF.RateLimitLower  SampleTimeMode=inherited  InitialCondition=Aactuator.LEF.IntegratorInitial
  LEF Saturation : Saturate  UpperLimit=Aactuator.LEF.AngleLimitUpper  LowerLimit=Aactuator.LEF.AngleLimitLower
  Square1 : Math  Operator=square  SignedPower=on  SaturateOnIntegerOverflow=on
  Sum : Sum  Inputs=-|+|+  InputSameDT=on  SaturateOnIntegerOverflow=on  OutDataTypeStr=Inherit: Same as first input
  Transfer Fcn : TransferFcn  Numerator=[2 7.25]  Denominator=[1 7.25]
  coeff1 : Constant  Value=1.45
  r2d2 : Gain  Gain=0.5  SaturateOnIntegerOverflow=on  OutDataTypeStr=Inherit: Same as input  ParamDataTypeStr=Inherit: Same as input
  r2d6 : Gain  Gain=9.05  SaturateOnIntegerOverflow=on  OutDataTypeStr=Inherit: Same as input  ParamDataTypeStr=Inherit: Same as input
  Out Bus Element3 : Outport  PortName=ActSensor_Out  Element=LEF_deg
  Out Bus Element2 : Outport  Port=2  PortName=ActPositions  Element=LEF_deg
  wires:
  Transfer Fcn/1 -> Gain2/1
  coeff1/1 -> Sum/3
  r2d6/1 -> Sum/1
  Square1/1 -> Divide2/1
  alpha (deg)/1 -> Transfer Fcn/1  "alpha (deg)"
  P (Pa)/1 -> Divide1/2
  vt (m/s)/1 -> Square1/1
  rho (kg/m^3)/1 -> Divide2/2  "rho(kg/m^3)"
  Divide1/1 -> r2d6/1
  Sum/1 -> LEF Saturation/1
  LEF Saturation/1 -> LEF Rate Limiter/1
  Divide2/1 -> r2d2/1
  r2d2/1 -> Divide1/1  "qbar (Pa)"
  Gain2/1 -> Sum/2
  LEF Rate Limiter/1 -> Out Bus Element2/1, Out Bus Element3/1

== system trimming/Vehicle/Propulsion/Actuators ==
  note: 初始值全部等於0和非0
      | 會影響模擬結果
  In Bus Element : Inport  PortName=Commands  Element=TVC_Z
  In Bus Element1 : Inport  PortName=Commands  Element=TVC_Y
  Gain4 : Gain  Gain=20.202  SaturateOnIntegerOverflow=on  OutDataTypeStr=Inherit: Same as input  ParamDataTypeStr=Inherit: Same as input
  Gain5 : Gain  Gain=20.202  SaturateOnIntegerOverflow=on  OutDataTypeStr=Inherit: Same as input  ParamDataTypeStr=Inherit: Same as input
  Rate Saturation4 : Saturate  UpperLimit=Aactuator.TVC_Z.RateLimitUpper  LowerLimit=Aactuator.TVC_Z.RateLimitLower
  Rate Saturation5 : Saturate  UpperLimit=Aactuator.TVC_Y.RateLimitUpper  LowerLimit=Aactuator.TVC_Y.RateLimitLower
  Sum4 : Sum  Inputs=|+-  InputSameDT=on  SaturateOnIntegerOverflow=on  OutDataTypeStr=Inherit: Same as first input
  Sum5 : Sum  Inputs=|+-  InputSameDT=on  SaturateOnIntegerOverflow=on  OutDataTypeStr=Inherit: Same as first input
  TVC_Y Integrator (degrees) : Integrator  InitialCondition=Aactuator.TVC_Y.IntegratorInitial  UpperSaturationLimit=30  LowerSaturationLimit=-30
  TVC_Y Saturation : Saturate  UpperLimit=Aactuator.TVC_Y.AngleLimitUpper  LowerLimit=Aactuator.TVC_Y.AngleLimitLower
  TVC_Z Integrator (degrees) : Integrator  InitialCondition=Aactuator.TVC_Z.IntegratorInitial  UpperSaturationLimit=30  LowerSaturationLimit=-30
  TVC_Z Saturation : Saturate  UpperLimit=Aactuator.TVC_Z.AngleLimitUpper  LowerLimit=Aactuator.TVC_Z.AngleLimitLower
  Out Bus Element : Outport  PortName=ActPositions  Element=TVC_Z_pitch_deg
  Out Bus Element1 : Outport  PortName=ActPositions  Element=TVC_Y_yaw_deg
  Out Bus Element2 : Outport  Port=2  PortName=ActSensor_Out  Element=TVC_Z_pitch_deg
  Out Bus Element3 : Outport  Port=2  PortName=ActSensor_Out  Element=TVC_Y_yaw_deg
  wires:
  Sum5/1 -> Gain5/1
  TVC_Y Saturation/1 -> Sum5/1
  TVC_Z Integrator (degrees)/1 -> Out Bus Element2/1, Out Bus Element/1, Sum4/2  "TVC_Z_pitch_deg"
  Sum4/1 -> Gain4/1
  In Bus Element1/1 -> TVC_Y Saturation/1  "Commands_TVC_Y_yaw"
  TVC_Y Integrator (degrees)/1 -> Out Bus Element3/1, Out Bus Element1/1, Sum5/2  "TVC_Y_yaw_deg"
  In Bus Element/1 -> TVC_Z Saturation/1  "Commands_TVC_Z_pitch"
  Rate Saturation5/1 -> TVC_Y Integrator (degrees)/1
  Gain4/1 -> Rate Saturation4/1
  Gain5/1 -> Rate Saturation5/1
  Rate Saturation4/1 -> TVC_Z Integrator (degrees)/1
  TVC_Z Saturation/1 -> Sum4/1

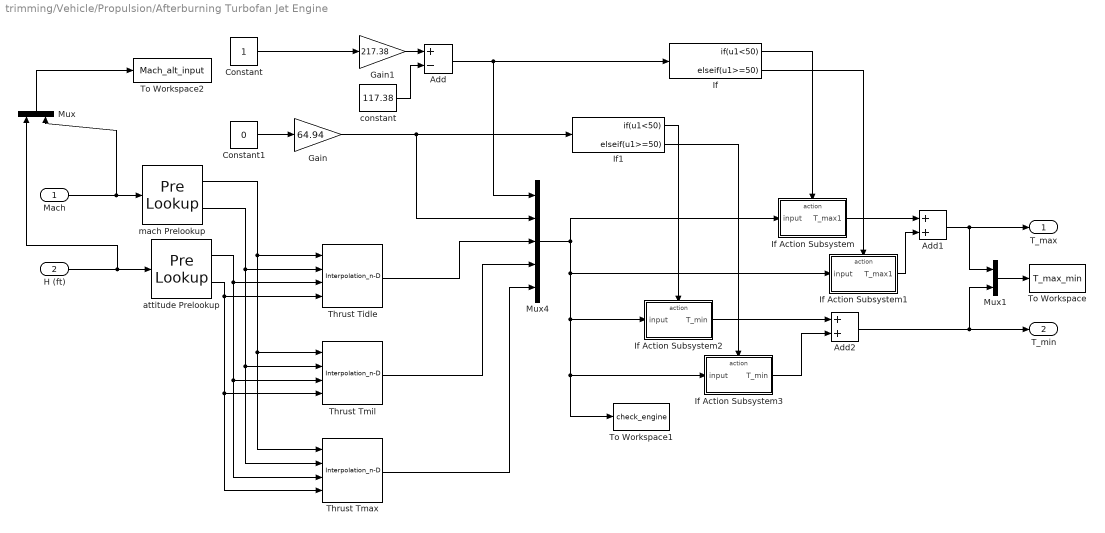
== system trimming/Vehicle/Propulsion/Afterburning Turbofan Jet Engine ==
  Mach : Inport
  H (ft) : Inport  Port=2
  Add : Sum  Inputs=+-
  Add1 : Sum
  Add2 : Sum
  Constant : Constant
  Constant1 : Constant  Value=0
  Gain : Gain  Gain=64.94
  Gain1 : Gain  Gain=217.38
  If : If  IfExpression=u1<50  ElseIfExpressions=u1>=50  ShowElse=off
  If Action Subsystem : Subsystem  TreatAsAtomicUnit=on
  If Action Subsystem1 : Subsystem  TreatAsAtomicUnit=on
  If Action Subsystem2 : Subsystem  TreatAsAtomicUnit=on
  If Action Subsystem3 : Subsystem  TreatAsAtomicUnit=on
  If1 : If  IfExpression=u1<50  ElseIfExpressions=u1>=50  ShowElse=off
  Mux : Mux  Inputs=2
  Mux1 : Mux  Inputs=2
  Mux4 : Mux  Inputs=5
  Thrust Tidle : Interpolation_n-D  Table=|  InternalRulePriority=Speed
      | [1060	670	880	1140	1500	1860
      | 635	425	690	1010	1330	1700
      | 60	25	345	755	1130	1525
      | -1020	-710	-300	350	910	1360
      | -2700	-1900	-1300	-247	600	1100
      | -3600	-1400	-595	-342	-200	700]
  Thrust Tmax : Interpolation_n-D  Table=reshape([20000,21420,22700,24240,26070,28886,15000,15700,16860,18910,21075,23319,10800,11225,12250,13760,15975,18300,7000,7323,8154,9285,11115,13484,4000,4435,5000,5700,6860,8642,2500,2600,2835,3215,3950,5057],6,6)  InternalRulePriority=Speed
  Thrust Tmil : Interpolation_n-D  Table=|  InternalRulePriority=Speed
      | [12680	9150	6200	3950	2450	1400
      | 12680	9150	6313	4040	2470	1400
      | 12610	9312	6610	4290	2600	1560
      | 12640	9839	7090	4660	2840	1660
      | 12390	10176	7750	5320	3250	1930
      | 11680	9848	8050	6100	3800	2310]
  To Workspace : ToWorkspace  VariableName=T_max_min  SaveFormat=Timeseries  SampleTime=-1
  To Workspace1 : ToWorkspace  VariableName=check_engine  SaveFormat=Timeseries  SampleTime=-1
  To Workspace2 : ToWorkspace  VariableName=Mach_alt_input  SaveFormat=Timeseries  SampleTime=-1
  attitude Prelookup : PreLookup  BreakpointsData=[0,10000,20000,30000,40000,50000]  IndexSearchMethod=Linear search  BeginIndexSearchUsingPreviousIndexResult=on  DiagnosticForOutOfRangeInput=Warning
  constant : Constant  Value=117.38
  mach Prelookup : PreLookup  BreakpointsData=[0,0.2,0.4,0.6,0.8,1]  IndexSearchMethod=Linear search  BeginIndexSearchUsingPreviousIndexResult=on  DiagnosticForOutOfRangeInput=Warning
  T_max : Outport  VectorParamsAs1DForOutWhenUnconnected=off
  T_min : Outport  Port=2  VectorParamsAs1DForOutWhenUnconnected=off
  wires:
  Mach/1 -> Mux/2, mach Prelookup/1
  H (ft)/1 -> attitude Prelookup/1, Mux/1
  Add2/1 -> T_min/1, Mux1/2
  Add1/1 -> T_max/1, Mux1/1
  attitude Prelookup/2 -> Thrust Tidle/4, Thrust Tmil/4, Thrust Tmax/4
  Mux1/1 -> To Workspace/1
  Thrust Tmil/1 -> Mux4/4
  Mux/1 -> To Workspace2/1
  Gain1/1 -> Add/1
  If Action Subsystem1/1(T_max1) -> Add1/2
  Constant/1 -> Gain1/1
  mach Prelookup/1 -> Thrust Tidle/1, Thrust Tmil/1, Thrust Tmax/1
  If/2 -> If Action Subsystem1/Action
  If1/2 -> If Action Subsystem3/Action
  If Action Subsystem3/1(T_min) -> Add2/2
  If Action Subsystem2/1(T_min) -> Add2/1
  If1/1 -> If Action Subsystem2/Action
  Gain/1 -> Mux4/2, If1/1
  If Action Subsystem/1(T_max1) -> Add1/1
  Thrust Tmax/1 -> Mux4/5
  mach Prelookup/2 -> Thrust Tidle/2, Thrust Tmil/2, Thrust Tmax/2
  Thrust Tidle/1 -> Mux4/3
  If/1 -> If Action Subsystem/Action
  Add/1 -> Mux4/1, If/1
  constant/1 -> Add/2
  Mux4/1 -> If Action Subsystem1/1("input "), If Action Subsystem2/1("input "), If Action Subsystem3/1("input "), To Workspace1/1, If Action Subsystem/1("input ")
  Constant1/1 -> Gain/1
  attitude Prelookup/1 -> Thrust Tidle/3, Thrust Tmil/3, Thrust Tmax/3

== system trimming/Vehicle/Propulsion/Thrust Vector Nozzle ZY ==
  note: pitching thrust Tz
  note: yawing thrust Ty
  note: axial thrust Tx
  T : Inport
  Actuator (deg) : Inport  Port=2
  " lt" : Inport  Port=3
  "+y, -r" : Gain
  "+y, -r1" : Gain  Gain=-1
  Angle Conversion : aerolibconvert2/Angle Conversion  IU=deg  OU=rad
  Angle Conversion1 : aerolibconvert2/Angle Conversion  IU=deg  OU=rad
  Bus Selector : BusSelector  OutputSignals=TVC_Z_pitch_deg,TVC_Y_yaw_deg
  Constant : Constant  Value=-1
  Cos : Trigonometry  Operator=cos
  Cos1 : Trigonometry  Operator=cos
  Mux1 : Mux  Inputs=6
  Product : Product  Inputs=3
  Product1 : Product  Inputs=4
  Product2 : Product
  Sin : Trigonometry
  Sin1 : Trigonometry
  pitch : Product
  rolling M : Constant  Value=0
  yaw : Product
  FM : Outport  VectorParamsAs1DForOutWhenUnconnected=off
  Tx : Outport  Port=2  VectorParamsAs1DForOutWhenUnconnected=off
  Ty : Outport  Port=3  VectorParamsAs1DForOutWhenUnconnected=off
  Tz : Outport  Port=4  VectorParamsAs1DForOutWhenUnconnected=off
  wires:
  rolling M/1 -> Mux1/4  "Mx"
  Product1/1 -> pitch/2, Tz/1, Mux1/3  "Tz"
  yaw/1 -> "+y, -r1"/1
  pitch/1 -> "+y, -r"/1
  "+y, -r1"/1 -> Mux1/6  "Mz"
  Product/1 -> Tx/1, Mux1/1  "Tx"
  T/1 -> Product1/2, Product2/1, Product/1  "T"
  " lt"/1 -> pitch/1, yaw/1  "lt"
  Product2/1 -> Ty/1, Mux1/2, yaw/2  "Ty"
  "+y, -r"/1 -> Mux1/5  "My"
  Mux1/1 -> FM/1
  Actuator (deg)/1 -> Bus Selector/1
  Bus Selector/1 -> Angle Conversion/1  "<TVC_Z_pitch_deg>"
  Bus Selector/2 -> Angle Conversion1/1  "<TVC_Y_yaw_deg>"
  Angle Conversion1/1 -> Sin1/1, Cos1/1
  Angle Conversion/1 -> Sin/1, Cos/1
  Cos/1 -> Product/2
  Cos1/1 -> Product1/4, Product/3
  Sin1/1 -> Product2/2
  Constant/1 -> Product1/1
  Sin/1 -> Product1/3

== system trimming/Vehicle/Actuators (no roll off)1/Engine block/If Action Subsystem ==
  note: Pow_max
      |
      | Pow_min
      |
      | T_idle
      |
      | T_mil
      |
      | T_max
  "input " : Inport
  Action Port : ActionPort
  Add : Sum
  Add1 : Sum  Inputs=-+
  Demux : Demux  Outputs=5
  Divide : Product  Inputs=**
  Gain : Gain  Gain=1/50
  Terminator : Terminator
  Terminator1 : Terminator
  T_max1 : Outport  VectorParamsAs1DForOutWhenUnconnected=off
  wires:
  Demux/3 -> Add1/1, Add/1
  Demux/4 -> Add1/2
  Add1/1 -> Divide/2
  Gain/1 -> Divide/1
  Divide/1 -> Add/2
  Add/1 -> T_max1/1
  "input "/1 -> Demux/1
  Demux/1 -> Gain/1
  Demux/2 -> Terminator/1
  Demux/5 -> Terminator1/1

== system trimming/Vehicle/Actuators (no roll off)1/Engine block/If Action Subsystem1 ==
  note: Pow_max
      |
      | Pow_min
      |
      | T_idle
      |
      | T_mil
      |
      | T_max
  "input " : Inport
  Action Port : ActionPort
  Add : Sum
  Add1 : Sum  Inputs=-+
  Add2 : Sum  Inputs=-+
  Constant : Constant  Value=50
  Demux : Demux  Outputs=5
  Gain : Gain  Gain=1/50
  Product : Product
  Terminator : Terminator
  Terminator1 : Terminator
  T_max1 : Outport  VectorParamsAs1DForOutWhenUnconnected=off
  wires:
  "input "/1 -> Demux/1
  Demux/4 -> Add/2, Add1/1
  Demux/5 -> Add1/2
  Demux/1 -> Add2/2
  Constant/1 -> Add2/1
  Add2/1 -> Gain/1
  Add1/1 -> Product/2
  Gain/1 -> Product/1
  Product/1 -> Add/1
  Add/1 -> T_max1/1
  Demux/3 -> Terminator1/1
  Demux/2 -> Terminator/1

== system trimming/Vehicle/Actuators (no roll off)1/Engine block/If Action Subsystem2 ==
  note: Pow_max
      |
      | Pow_min
      |
      | T_idle
      |
      | T_mil
      |
      | T_max
  "input " : Inport
  Action Port : ActionPort
  Add : Sum
  Add1 : Sum  Inputs=-+
  Demux : Demux  Outputs=5
  Divide : Product  Inputs=**
  Gain : Gain  Gain=1/50
  Terminator : Terminator
  Terminator1 : Terminator
  T_min : Outport  VectorParamsAs1DForOutWhenUnconnected=off
  wires:
  Demux/3 -> Add1/1, Add/1
  Demux/4 -> Add1/2
  Add1/1 -> Divide/2
  Gain/1 -> Divide/1
  Divide/1 -> Add/2
  Add/1 -> T_min/1
  "input "/1 -> Demux/1
  Demux/2 -> Gain/1
  Demux/5 -> Terminator1/1
  Demux/1 -> Terminator/1

== system trimming/Vehicle/Actuators (no roll off)1/Engine block/If Action Subsystem3 ==
  note: Pow_max
      |
      | Pow_min
      |
      | T_idle
      |
      | T_mil
      |
      | T_max
  "input " : Inport
  Action Port : ActionPort
  Add : Sum
  Add1 : Sum  Inputs=-+
  Add2 : Sum  Inputs=-+
  Constant : Constant  Value=50
  Demux : Demux  Outputs=5
  Gain : Gain  Gain=1/50
  Product : Product
  Terminator : Terminator
  Terminator1 : Terminator
  T_min : Outport  VectorParamsAs1DForOutWhenUnconnected=off
  wires:
  "input "/1 -> Demux/1
  Demux/4 -> Add/2, Add1/1
  Demux/5 -> Add1/2
  Constant/1 -> Add2/1
  Add2/1 -> Gain/1
  Add1/1 -> Product/2
  Gain/1 -> Product/1
  Product/1 -> Add/1
  Add/1 -> T_min/1
  Demux/3 -> Terminator1/1
  Demux/2 -> Add2/2
  Demux/1 -> Terminator/1

== system trimming/Vehicle/Aerodynamics/Aerofynamic Coefficients/CXT ==
  note: 氣動力表格僅提供到攻角到
      | 45度，超過45度後皆採用45
      | 度的氣動力係數
  alpha (deg) : Inport
  "beta (deg) " : Inport  Port=2
  elevator (deg) : Inport  Port=3
  dlef : Inport  Port=4
  qc_2v : Inport  Port=5
  sb : Inport  Port=6
  Add : Sum  Inputs=+-
  Add1 : Sum  Inputs=++++
  Add2 : Sum
  Cx : Interpolation_n-D  NumberOfTableDimensions=3  Table=AeroCoeff.Cx
      settings: InputPortMap=u0,u1,u2,u3,u4,u5
  Cx_elevator0 : Interpolation_n-D  Table=AeroCoeff.Cx_elevator0
  Cx_lef : Interpolation_n-D  Table=AeroCoeff.Cx_lef
  "Cx_q " : Interpolation_n-D  NumberOfTableDimensions=1  Table=AeroCoeff.Cx_q
      settings: InputPortMap=u0,u1
  Cx_q_lef : Interpolation_n-D  NumberOfTableDimensions=1  Table=AeroCoeff.Cx_q_lef
      settings: InputPortMap=u0,u1
  Product{,1..3} (4 alike) : Product
  alpha Prelookup : PreLookup  BreakpointsData=[-20,-15,-10,-5,0,5,10,15,20,25,30,35,40,45,50,55,60,70,80,90]  IndexSearchMethod=Linear search  BeginIndexSearchUsingPreviousIndexResult=on  DiagnosticForOutOfRangeInput=Warning
  beta Prelookup : PreLookup  BreakpointsData=[-30,-25,-20,-15,-10,-8,-6,-4,-2,0,2,4,6,8,10,15,20,25,30]  IndexSearchMethod=Linear search  BeginIndexSearchUsingPreviousIndexResult=on  DiagnosticForOutOfRangeInput=Warning
  dCX_sb : Interpolation_n-D  NumberOfTableDimensions=1  Table=AeroCoeff.dCX_sb
      settings: InputPortMap=u0,u1
  elevator Prelookup : PreLookup  BreakpointsData=[-25 -10 0 10 25]  IndexSearchMethod=Linear search  BeginIndexSearchUsingPreviousIndexResult=on  DiagnosticForOutOfRangeInput=Warning
  Cx_tot : Outport  VectorParamsAs1DForOutWhenUnconnected=off
  wires:
  beta Prelookup/2 -> Cx_elevator0/4, Cx_lef/4, Cx/4
  beta Prelookup/1 -> Cx_elevator0/3, Cx_lef/3, Cx/3
  Cx_lef/1 -> Add/1
  alpha Prelookup/1 -> Cx_q_lef/1, dCX_sb/1, "Cx_q "/1, Cx_elevator0/1, Cx/1, Cx_lef/1
  elevator Prelookup/2 -> Cx/6
  elevator (deg)/1 -> elevator Prelookup/1
  "beta (deg) "/1 -> beta Prelookup/1
  Add/1 -> Product/1
  alpha Prelookup/2 -> Cx_q_lef/2, dCX_sb/2, "Cx_q "/2, Cx_elevator0/2, Cx_lef/2, Cx/2
  Product/1 -> Add1/2
  elevator Prelookup/1 -> Cx/5
  Add2/1 -> Product2/1
  Cx/1 -> Add1/1
  Cx_elevator0/1 -> Add/2
  Cx_q_lef/1 -> Product1/1
  Product1/1 -> Add2/2
  "Cx_q "/1 -> Add2/1
  dlef/1 -> Product/2, Product1/2
  Product2/1 -> Add1/3
  Add1/1 -> Cx_tot/1
  qc_2v/1 -> Product2/2
  dCX_sb/1 -> Product3/1
  sb/1 -> Product3/2
  Product3/1 -> Add1/4
  alpha (deg)/1 -> alpha Prelookup/1
